simulink model "AEB_Project"  (R2024b)
settings: Solver=ode4  StartTime=0.0  StopTime=Tsim  FixedStep=Ts  RelTol=1e-3
values from neighbouring files (symbols this model uses):
  a_cmd_test = 0    [init_AEB.m]
  a_full = -6.0    (= -6)    [init_AEB.m]
  a_max = 2.0    (= 2)    [init_AEB.m]
  v_ego0 = 20    [init_AEB.m]
  v_target0 = 0    [init_AEB.m]
  x_ego0 = 0    [init_AEB.m]
  x_target0 = 100    [init_AEB.m]
settings Model: Creator=jun_mac  LastModifiedBy=jun_mac

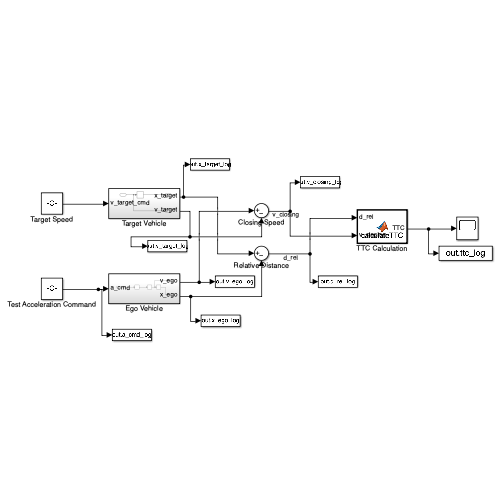
[thumbnail: Simulink's stored preview of the top-level diagram]
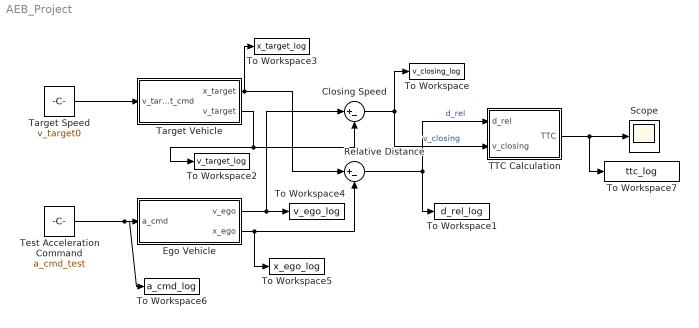
== system AEB_Project ==
  Closing Speed : Sum  Inputs=|+-
  Ego Vehicle : Subsystem
  Relative Distance : Sum  Inputs=|+-
  Scope : Scope
  TTC Calculation : MATLAB Function  TreatAsAtomicUnit=on
  Target Speed : Constant  Value=v_target0
  Target Vehicle : Subsystem
  Test Acceleration Command : Constant  Value=a_cmd_test
  To Workspace : ToWorkspace  VariableName=v_closing_log  SaveFormat=Timeseries  SampleTime=-1
  To Workspace1 : ToWorkspace  VariableName=d_rel_log  SaveFormat=Timeseries  SampleTime=-1
  To Workspace2 : ToWorkspace  VariableName=v_target_log  SaveFormat=Timeseries  SampleTime=-1
  To Workspace3 : ToWorkspace  VariableName=x_target_log  SaveFormat=Timeseries  SampleTime=-1
  To Workspace4 : ToWorkspace  VariableName=v_ego_log  SaveFormat=Timeseries  SampleTime=-1
  To Workspace5 : ToWorkspace  VariableName=x_ego_log  SaveFormat=Timeseries  SampleTime=-1
  To Workspace6 : ToWorkspace  VariableName=a_cmd_log  SaveFormat=Timeseries  SampleTime=-1
  To Workspace7 : ToWorkspace  VariableName=ttc_log  SaveFormat=Timeseries  SampleTime=-1
  wires:
  Target Speed/1 -> Target Vehicle/1(v_target_cmd)
  Test Acceleration Command/1 -> To Workspace6/1, Ego Vehicle/1(a_cmd)
  Target Vehicle/1(x_target) -> To Workspace3/1, Relative Distance/1
  Ego Vehicle/2(x_ego) -> To Workspace5/1, Relative Distance/2
  Relative Distance/1 -> TTC Calculation/1(d_rel), To Workspace1/1  "d_rel"
  Ego Vehicle/1(v_ego) -> To Workspace4/1, Closing Speed/1
  Target Vehicle/2(v_target) -> To Workspace2/1, Closing Speed/2
  Closing Speed/1 -> TTC Calculation/2(v_closing), To Workspace/1  "v_closing"
  TTC Calculation/1(TTC) -> To Workspace7/1, Scope/1

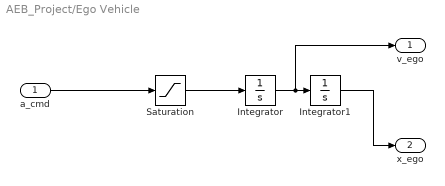
== system AEB_Project/Ego Vehicle ==
  a_cmd : Inport
  Integrator : Integrator  InitialCondition=v_ego0  LimitOutput=on  UpperSaturationLimit=50  LowerSaturationLimit=0
  Integrator1 : Integrator  InitialCondition=x_ego0
  Saturation : Saturate  UpperLimit=a_max  LowerLimit=a_full
  v_ego : Outport
  x_ego : Outport  Port=2
  wires:
  a_cmd/1 -> Saturation/1
  Saturation/1 -> Integrator/1
  Integrator/1 -> v_ego/1, Integrator1/1
  Integrator1/1 -> x_ego/1

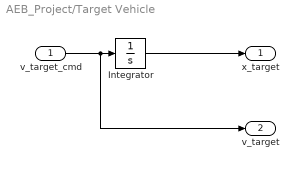
== system AEB_Project/Target Vehicle ==
  v_target_cmd : Inport
  Integrator : Integrator  InitialCondition=x_target0
  x_target : Outport
  v_target : Outport  Port=2
  wires:
  v_target_cmd/1 -> v_target/1, Integrator/1
  Integrator/1 -> x_target/1

== matlab function AEB_Project/TTC Calculation ==
  data: d_rel input; TTC output; v_closing input
function TTC = calculateTTC(d_rel, v_closing)
%#codegen

% AEB Time To Collision calculation

if d_rel <= 0

    % Collision already occurred
    TTC = 0;

elseif v_closing > 0.1

    % Ego vehicle is approaching the target
    TTC = d_rel / v_closing;

else

    % No meaningful collision risk
    TTC = 99;

end
